simulink model "PIDtuning"  (R2023a)
settings: Solver=VariableStepAuto  StartTime=0.0  StopTime=20  RelTol=1e-3
libraries: slpidlib x1
settings Model: Creator=hwayoungkim  LastModifiedBy=hwayoungkim

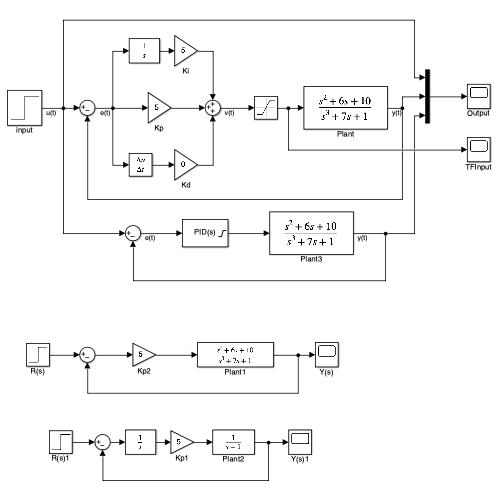
[thumbnail: Simulink's stored preview of the top-level diagram]
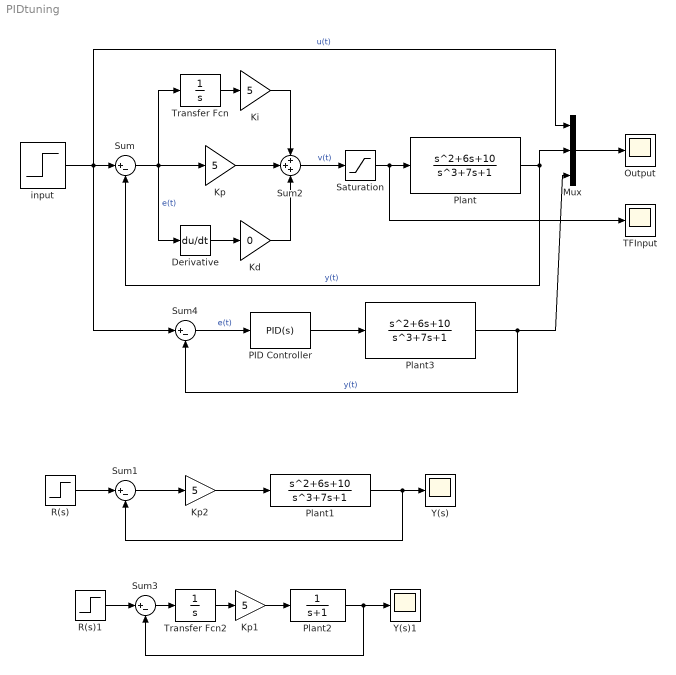
== system PIDtuning ==
  Derivative : Derivative
  Kd : Gain  Gain=0
  Ki : Gain  Gain=5
  Kp : Gain  Gain=5
  Kp1 : Gain  Gain=5
  Kp2 : Gain  Gain=5
  Mux : Mux  Inputs=3
  Output : Scope
  PID Controller : slpidlib/PID Controller  Controller=PID  Form=Parallel  TimeDomain=Continuous-time  UseExternalTs=off  SampleTime=-1  IntegratorMethod=Forward Euler  FilterMethod=Forward Euler  ControllerParametersSource=internal  P=5  I=5  UseKiTs=off  D=0  N=100  UseFilter=on  TunerSelectOption=Transfer Function Based (PID Tuner App)  InitialConditionSource=internal  InitialConditionForIntegrator=0  InitialConditionForFilter=0  DifferentiatorICPrevScaledInput=0  ExternalReset=none  TrackingMode=off  Kt=1  LimitOutput=on  SatLimitsSource=internal  UpperSaturationLimit=2  LowerSaturationLimit=-2  LinearizeAsGain=off  AntiWindupMode=none  Kb=1  LimitIntegrator=off  UpperIntegratorSaturationLimit=inf  LowerIntegratorSaturationLimit=-inf  POutMin=[]  POutMax=[]  IOutMin=[]  IOutMax=[]  DOutMin=[]  DOutMax=[]  NOutMin=[]  NOutMax=[]  SumOutMin=[]  SumOutMax=[]  SaturationOutMin=[]  SaturationOutMax=[]  PParamMin=[]  PParamMax=[]  IParamMin=[]  IParamMax=[]  DParamMin=[]  DParamMax=[]  NParamMin=[]  NParamMax=[]  KbParamMin=[]  KbParamMax=[]  KtParamMin=[]  KtParamMax=[]  KbOutMin=[]  KbOutMax=[]  KtOutMin=[]  KtOutMax=[]  IntegratorOutMin=[]  IntegratorOutMax=[]  FilterOutMin=[]  FilterOutMax=[]  SumI1OutMin=[]  SumI1OutMax=[]  SumI2OutMin=[]  SumI2OutMax=[]  SumI3OutMin=[]  SumI3OutMax=[]  SumI4OutMin=[]  SumI4OutMax=[]  SumDOutMin=[]  SumDOutMax=[]  DifferentiatorOutMin=[]  DifferentiatorOutMax=[]  FilterDiffOutCoefMin=[]  FilterDiffOutCoefMax=[]  ReciprocalOutMin=[]  ReciprocalOutMax=[]  SumDenOutMin=[]  SumDenOutMax=[]  SumNumOutMin=[]  SumNumOutMax=[]  DivideOutMin=[]  DivideOutMax=[]  UdiffTsProdOutMin=[]  UdiffTsProdOutMax=[]  NTsProdOutMin=[]  NTsProdOutMax=[]  UintegralTsProdOutMin=[]  UintegralTsProdOutMax=[]  UngainTsProdOutMin=[]  UngainTsProdOutMax=[]  ClampingZeroOutDataTypeStr=Inherit: Inherit via back propagation  ClampingZeroOutMin=[]  ClampingZeroOutMax=[]  FilterDenConstantOutDataTypeStr=Inherit: Inherit via back propagation  FilterDenConstantOutMin=[]  FilterDenConstantOutMax=[]  PCopyOutDataTypeStr=Inherit: Inherit via back propagation  PCopyOutMin=[]  PCopyOutMax=[]  NCopyOutDataTypeStr=Inherit: Inherit via back propagation  NCopyOutMin=[]  NCopyOutMax=[]  IntegratorContinuousStateAttributes=''  IntegratorStateMustResolveToSignalObject=off  IntegratorRTWStateStorageClass=Auto  FilterContinuousStateAttributes=''  FilterStateMustResolveToSignalObject=off  FilterRTWStateStorageClass=Auto  ParallelPVariant=InternalParameters  IdealPVariant=Disabled  IVariant=InternalParameters  DVariant=InternalParameters  IntegratorVariant=Continuous  SatVariant=Enabled  AWVariant=Passthrough  PCopyVariant=Disabled  TRVariant=Disabled  FdbkBlocksVariant=Forward  IdealPFdbkVariant=Disabled  SatFdbkVariant=Disabled  DerivativeFilterVariant=ContFilter  NVariant=InternalParameters  NCopyVariant=Disabled  FilterICVariant=InternalICsFilter  IntegratorICVariant=InternalICs  ExternalResetVariant=Disabled  TRSumVariant=Passthrough  SumFdbkVariant=Disabled  SumVariant=Sum_PID  TsampFilterVariant=InternalTs  TsampNgainVariant=Passthrough  TsampIntegralVariant=Disabled_SignalSpec  ExternalSaturationOutDataTypeStr=Inherit: Same as second input
  Plant : TransferFcn  Numerator=[1 6 10]  Denominator=[1 0 7 1]
  Plant1 : TransferFcn  Numerator=[1 6 10]  Denominator=[1 0 7 1]
  Plant2 : TransferFcn  Denominator=[1 1]
  Plant3 : TransferFcn  Numerator=[1 6 10]  Denominator=[1 0 7 1]
  R(s) : Step  SampleTime=0
  R(s)1 : Step  SampleTime=0
  Saturation : Saturate  UpperLimit=2  LowerLimit=-2
  Sum{,1,3..4} (4 alike) : Sum  Inputs=|+-
  Sum2 : Sum  Inputs=+++
  TFInput : Scope
  Transfer Fcn : TransferFcn  Denominator=[1 0]
  Transfer Fcn2 : TransferFcn  Denominator=[1 0]
  Y(s) : Scope
  Y(s)1 : Scope
  input : Step  After=5  SampleTime=0
  wires:
  Sum/1 -> Derivative/1, Transfer Fcn/1, Kp/1  "e(t)"
  input/1 -> Sum4/1, Sum/1, Mux/1  "u(t)"
  R(s)/1 -> Sum1/1
  Mux/1 -> Output/1
  Plant/1 -> Sum/2, Mux/2  "y(t)"
  Plant1/1 -> Sum1/2, Y(s)/1
  Transfer Fcn/1 -> Ki/1
  Sum2/1 -> Saturation/1  "v(t)"
  Ki/1 -> Sum2/1
  Kp/1 -> Sum2/2
  Kp2/1 -> Plant1/1
  Sum1/1 -> Kp2/1
  Kp1/1 -> Plant2/1
  Sum3/1 -> Transfer Fcn2/1
  Plant2/1 -> Sum3/2, Y(s)1/1
  R(s)1/1 -> Sum3/1
  Transfer Fcn2/1 -> Kp1/1
  Derivative/1 -> Kd/1
  Kd/1 -> Sum2/3
  Saturation/1 -> TFInput/1, Plant/1
  Sum4/1 -> PID Controller/1  "e(t)"
  PID Controller/1 -> Plant3/1
  Plant3/1 -> Mux/3, Sum4/2  "y(t)"
